simulink model "communication"  (R2025b)
settings: Solver=FixedStepAuto  StartTime=0.0  StopTime=1  FixedStep=0.01  RelTol=1e-3
undefined symbols (not defined in the file or in its folder): LF
libraries: instrumentseriallib x1, arduinolib x1
settings Model: ExtModeTrigDuration=2  Creator=CoolA  LastModifiedBy=root
settings SolverCC: AutoInsertRateTranBlk=on
settings OptimizationCC: EnhancedBackFolding=on  PassReuseOutputArgsAs=Individual arguments  ZeroExternalMemoryAtStartup=off  ZeroInternalMemoryAtStartup=off  MaxStackSize=64  OptimizeBlockOrder=speed  DifferentSizesBufferReuse=on  OptimizationCustomize=off  EfficientTunableParamExpr=on
settings DebuggingCC: ParameterTunabilityLossMsg=error
settings HardwareCC: ProdBitPerInt=16.0  ProdBitPerPointer=16.0  ProdBitPerSizeT=16.0  ProdBitPerPtrDiffT=16.0  ProdLargestAtomicFloat=None  ProdWordSize=8.0  ProdHWDeviceType=Atmel->AVR  UseEmbeddedCoderFeatures=off  UseSimulinkCoderFeatures=off
settings RTWCC: SystemTargetFile=ert.tlc  HardwareBoard=Arduino Uno  TemplateMakefile=ert_default_tmf  Toolchain=Arduino AVR  Description=Embedded Coder
settings CodeAppCC: ForceParamTrailComments=on  IgnoreCustomStorageClasses=off  OperatorAnnotations=on  SimulinkDataObjDesc=on  SFDataObjDesc=on  InsertBlockDesc=on
settings ERTTargetCC: ExtModeTransport=3.0  ExtModeStaticAlloc=on  ExtModeAutomaticAllocSize=off  ExtModeStaticAllocSize=250.0  ExtModeMexFile=ext_xcp  ExtModeIntrfLevel=Level2 - Open  InlinedParameterPlacement=Hierarchical  SupportContinuousTime=on  SupportNonInlinedSFcns=on  SupportVariableSizeSignals=on

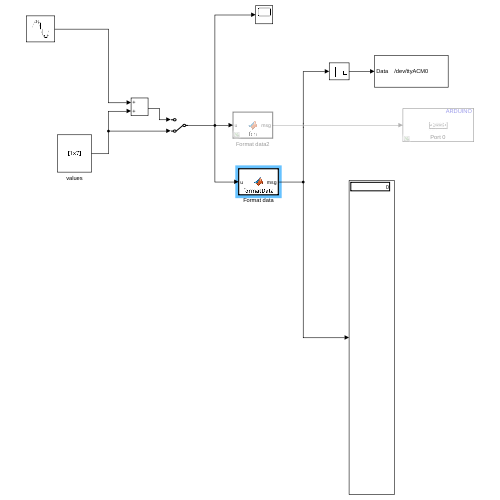
[thumbnail: Simulink's stored preview of the top-level diagram]
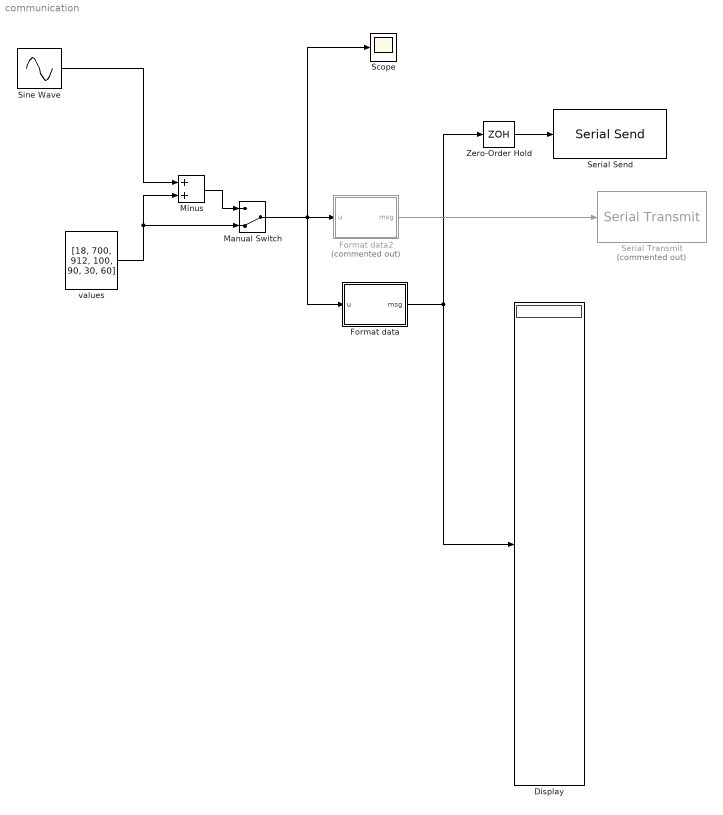
== system communication ==
  Display : Display
  Format data : MATLAB Function  TreatAsAtomicUnit=on
  Format data2 : MATLAB Function  Commented=on  TreatAsAtomicUnit=on
  Manual Switch : ManualSwitch  CurrentSetting=0
  Minus : Sum
  Scope : Scope
      settings: ActiveDisplayYMinimum=-106.24996750052651  ActiveDisplayYMaximum=1036.2499928659679
  Serial Send : instrumentseriallib/Serial Send  Priority=1  PortSel=/dev/ttyACM0  Port=/dev/ttyACM0  ComPort=/dev/ttyACM0  Header=[]  Terminator=LF ('\n')  CustomTerminator=[]  EnableBlockingMode=on  SimulateUsing=Interpreted execution  BlockInModel=on  aMode=1
  Serial Transmit : arduinolib/Serial Transmit  Commented=on  portNumber=0  sendmode=println  sendformat=Decimal  floatprecision=2  header=[]  terminator=[]  blockPlatform=ARDUINO
  Sine Wave : Sin  Amplitude=ones(7,1)*10  Bias=zeros(7,1)  SampleTime=0.01
  Zero-Order Hold : ZeroOrderHold  SampleTime=-1
  values : Constant  Value=[18, 700, 912, 100, 90, 30, 60]
  wires:
  values/1 -> Manual Switch/2, Minus/2
  Manual Switch/1 -> Scope/1, Format data2/1(u), Format data/1(u)
  Format data/1(msg) -> Display/1, Zero-Order Hold/1
  Sine Wave/1 -> Minus/1
  Format data2/1(msg) -> Serial Transmit/1
  Minus/1 -> Manual Switch/1
  Zero-Order Hold/1 -> Serial Send/1

== matlab function communication/Format data ==
  data: u input; msg output uint8 size=[1 29]
% function msg = fcn(u)
% MAX_LEN = 30;
% u = int8(u);
% msg = sprintf('<%03d,%03d,%03d,%03d,%03d,%03d,%03d>\n', u(1), u(2), u(3), u(4), u(5), u(6), u(7));
% 
% % 03 ensures 3 digits

function msg = formatData(u)
%#codegen

MAX_LEN = 29;
msg = uint8(zeros(1, MAX_LEN));

u = int16(u);

str = sprintf('<%03d,%03d,%03d,%03d,%03d,%03d,%03d>', ...
    u(1), u(2), u(3), u(4), u(5), u(6), u(7));

len = min(length(str), MAX_LEN);
msg(1:len) = uint8(str(1:len));

== matlab function communication/Format data2 ==
  data: u input; msg output string
function msg = fcn(u)
msg = sprintf('<%03d,%03d,%03d,%03d,%03d,%03d,%03d>', ...
    u(1), u(2), u(3), u(4), u(5), u(6), u(7));
